simulink model "learning"  (R2021a)
settings: Solver=VariableStepAuto  StartTime=0.0  StopTime=1.5  RelTol=1e-3
undefined symbols (not defined in the file): Radix
libraries: dspswit3 x4, dspxfrm3 x3, dspstat3 x2, visionstatistics x1, dspindex x1, dspsigops x1
settings Model: Creator=DAO1WA2  LastModifiedBy=O Darwish
settings SolverCC: AlgebraicLoopSolver=TrustRegion
settings DebuggingCC: SFMachineParentedDataDiag=warning

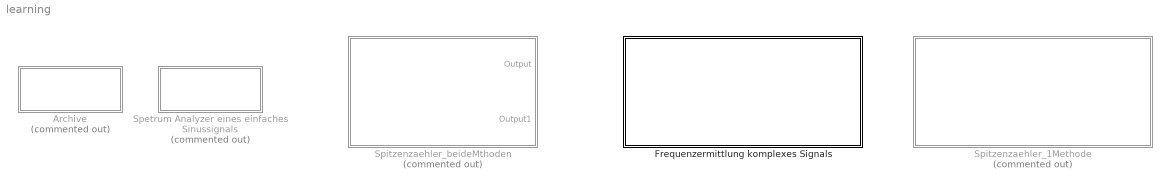
== system learning ==
  Archive : Subsystem  Commented=on
  Frequenzermittlung komplexes Signals : Subsystem
  Spetrum Analyzer eines einfaches Sinussignals : Subsystem  Commented=on
  Spitzenzaehler_1Methode : Subsystem  Commented=on
  Spitzenzaehler_beideMthoden : Subsystem  Commented=on

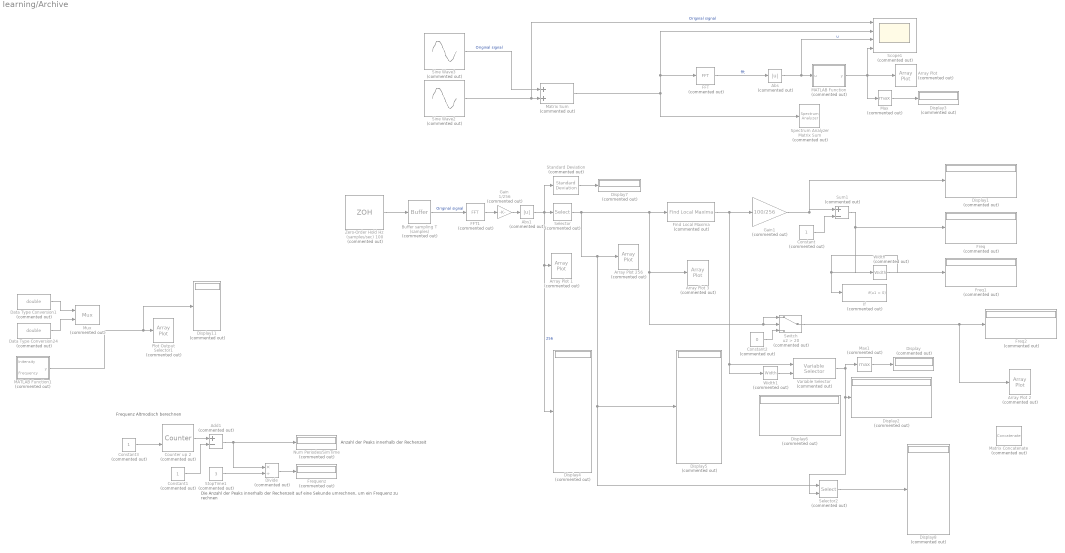
== system learning/Archive ==
  note: Frequenz Altmodisch berechnen
  note: Die Anzahl der Peaks innerhalb der Rechenzeit auf eine Sekunde umrechnen, um ein Frequenz zu rechnen
  note: Anzahl der Peaks innerhalb der Rechenzeit
  Abs : Abs  Commented=on
  Abs1 : Abs  Commented=on
  Add1 : Sum  Commented=on  Inputs=+-
  Array Plot : ArrayPlot  Commented=on  WindowPosition=[1925.8 897 1920 1095.2]  AxesScaling=Manual  YLimits=[89.0635,109.063]  ShowLegend=on  DefaultConfigurationName=dsp.scopes.ArrayPlotBlockSpecification
  Array Plot 1 : ArrayPlot  Commented=on  WindowPosition=[1.8 32.2 1532.8 748.8]  AxesScaling=Manual  YLimits=[-12.1535,116.039]  DefaultConfigurationName=dsp.scopes.ArrayPlotBlockSpecification
  Array Plot 2 : ArrayPlot  Commented=on  WindowPosition=[2 32.2 1532.8 748.8]  AxesScaling=Manual  YLimits=[-11.2764,109.153]  DefaultConfigurationName=dsp.scopes.ArrayPlotBlockSpecification
  Array Plot 256 : ArrayPlot  Commented=on  WindowPosition=[1.8 32.2 1532.8 748.8]  AxesScaling=Manual  YLimits=[-11.2764,109.153]  DefaultConfigurationName=dsp.scopes.ArrayPlotBlockSpecification
  Array Plot 3 : ArrayPlot  Commented=on  WindowPosition=[2.6 33 1532.8 748.8]  AxesScaling=Manual  YLimits=[-11.2764,109.153]  DefaultConfigurationName=dsp.scopes.ArrayPlotBlockSpecification
  Buffer sampling T (samples) : Buffer  Commented=on  N=256  V=128  OutputFrames=off
  Constant : Constant  Commented=on
  Constant1 : Constant  Commented=on
  Constant2 : Constant  Commented=on  Value=0
  Constant3 : Constant  Commented=on
  Counter up 2 : dspswit3/Counter  Commented=on  Direction=Up  CountEvent=Rising edge  CounterSize=User defined  MaxCount=255  InitialCount=0  Output=Count  HitValue=32  ResetInput=on  SamplesPerFrame=1  Ts=1  CntDtype=double  HitDtype=Logical
  Data Type Conversion1 : DataTypeConversion  Commented=on  OutDataTypeStr=double  RndMeth=Zero
  Data Type Conversion24 : DataTypeConversion  Commented=on  OutDataTypeStr=double  RndMeth=Zero
  Display{,1..8,11} (10 alike) : Display  Commented=on
  Divide : Product  Commented=on  Inputs=*/
  FFT : dspxfrm3/FFT  Commented=on  FFTImplementation=Auto  CompMethod=Table lookup  TableOpt=NEW  TableOptActive=Speed  BitRevOrder=off  Normalize=on  InheritFFTLength=on  FFTLength=64  WrapInput=on  roundingMode=Floor  overflowMode=off  firstCoeffDataTypeStr=Inherit: Same word length as input  firstCoeffLastDataTypeStr=Inherit: Same word length as input  outputMin=[]  outputMax=[]
  FFT1 : dspxfrm3/FFT  Commented=on  FFTImplementation=Radix-2  CompMethod=Table lookup  TableOpt=NEW  TableOptActive=Speed  BitRevOrder=off  Normalize=off  InheritFFTLength=on  FFTLength=256  WrapInput=off  roundingMode=Floor  overflowMode=off  firstCoeffDataTypeStr=Inherit: Same word length as input  firstCoeffLastDataTypeStr=Inherit: Same word length as input  outputMin=[]  outputMax=[]
  Find Local Maxima : visionstatistics/Find Local Maxima  Commented=on  num_peaks=4  nhood_size=[9 1]  src_thresh=Obsolete9b  src_thresh_inuse=Specify via dialog  threshold=10  inputIsHough=off  dt_peak=double  isOutVarDim=on  dt_count=double
      settings: SourceProductBaseCode=VP
  Freq : Display  Commented=on
  Freq1 : Display  Commented=on
  Freq2 : Display  Commented=on
  Frequenz : Display  Commented=on
  Gain : Gain  Commented=on  Gain=1/256
  Gain1 : Gain  Commented=on  Gain=100/256
  If : If  Commented=on  ShowElse=off
  MATLAB Function : MATLAB Function  Commented=on  TreatAsAtomicUnit=on
  MATLAB Function1 : MATLAB Function  Commented=on  TreatAsAtomicUnit=on
  Matrix Concatenate : Concatenate  Commented=on  NumInputs=1  Mode=Multidimensional array
  Matrix Sum : Sum  Commented=on
  Max : MinMax  Commented=on  Function=max
  Max1 : MinMax  Commented=on  Function=max
  Mux : Mux  Commented=on  Inputs=2
      settings: DisplayOption=signals
  Num Periodes/SimTime : Display  Commented=on
  Plot Output Selector1 : ArrayPlot  Commented=on  WindowPosition=[1 31.4 1536 758.4]  AxesScaling=Manual  YLimits=[-12.0102,109.123]  DefaultConfigurationName=dsp.scopes.ArrayPlotBlockSpecification
  Scope1 : Scope  Commented=on  NumInputPorts=4
  Selector : Selector  Commented=on  IndexOptions=Index vector (dialog)  Indices=1:128  OutputSizes=1
  Selector2 : Selector  Commented=on  IndexMode=Zero-based  IndexOptions=Index vector (port)  Indices=[1 3]  OutputSizes=1
  Sine Wave2 : Sin  Commented=on  Amplitude=325  Frequency=200  Samples=100  SampleTime=0.0001
  Sine Wave3 : Sin  Commented=on  SineType=Sample based  Amplitude=325  Frequency=314  Samples=100  SampleTime=0.0001
  Spectrum Analyzer Matrix Sum : SpectrumAnalyzer  Commented=on
  Standard Deviation : dspstat3/Standard Deviation  Commented=on  run=off  directionMode=Each column  dimension=1  InputProcessing=Columns as channels (frame based)  reset_popup=None  roiEnable=off  roiType=Rectangles  roiPortion=Entire ROI  roiOutput=Individual statistics for each ROI  roiFlag=off
      settings: SourceProductBaseCode=DS
  StopTime1 : Constant  Commented=on  Value=3
  Sum1 : Sum  Commented=on  Inputs=|+-
  Switch : Switch  Commented=on  Criteria=u2 > Threshold  Threshold=20
  Variable Selector : dspindex/Variable Selector  Commented=on  NumInputs=1  rowsOrCols=Columns  IdxMode=Variable  Elements=[1 3]  ZerOneIdxMode=One-based  errmode=Clip Index  FillMode=off  FillValues=0
  Width : Width  Commented=on
  Width1 : Width  Commented=on
  Zero-Order Hold Hz (samples/sec) 100 : ZeroOrderHold  Commented=on  SampleTime=1e-2
  wires:
  FFT/1 -> Abs/1  "fft"
  MATLAB Function1/1(y) -> Display11/1, Plot Output Selector1/1
  Divide/1 -> Frequenz/1
  Gain1/1 -> Display1/1, Sum1/1
  Selector/1 -> Find Local Maxima/1, Array Plot 3/1, Switch/1, Switch/2, Display5/1, Selector2/1, Array Plot 256/1
  Standard Deviation/1 -> Display7/1
  Constant2/1 -> Switch/3
  MATLAB Function/1(y) -> Scope1/4, Max/1, Array Plot/1
  Data Type Conversion1/1 -> Mux/1
  Width1/1 -> Variable Selector/2
  Switch/1 -> Array Plot 2/1, Freq2/1
  Max/1 -> Display3/1
  Sum1/1 -> Width/1, Freq/1
  Max1/1 -> Display/1
  Width/1 -> If/1, Freq1/1
  Constant/1 -> Sum1/2
  Variable Selector/1 -> Selector2/2, Display2/1, Max1/1
  Abs1/1 -> Array Plot 1/1, Display4/1, Standard Deviation/1, Selector/1  "256"
  Gain/1 -> Abs1/1
  Buffer sampling T (samples)/1 -> FFT1/1  "Original signal"
  FFT1/1 -> Gain/1
  Selector2/1 -> Display8/1
  Find Local Maxima/1 -> Width1/1, Variable Selector/1, Gain1/1
  Data Type Conversion24/1 -> Mux/2
  Constant1/1 -> Add1/2
  Zero-Order Hold Hz (samples/sec) 100/1 -> Buffer sampling T (samples)/1
  Sine Wave3/1 -> Matrix Sum/1  "Original signal"
  Add1/1 -> Divide/1, Num Periodes/SimTime/1
  Abs/1 -> Scope1/3, MATLAB Function/1(u)  "u"
  StopTime1/1 -> Divide/2
  Counter up 2/1 -> Add1/1
  Matrix Sum/1 -> FFT/1, Scope1/2, Spectrum Analyzer Matrix Sum/1
  Constant3/1 -> Counter up 2/2
  Sine Wave2/1 -> Scope1/1, Matrix Sum/2  "Original signal"

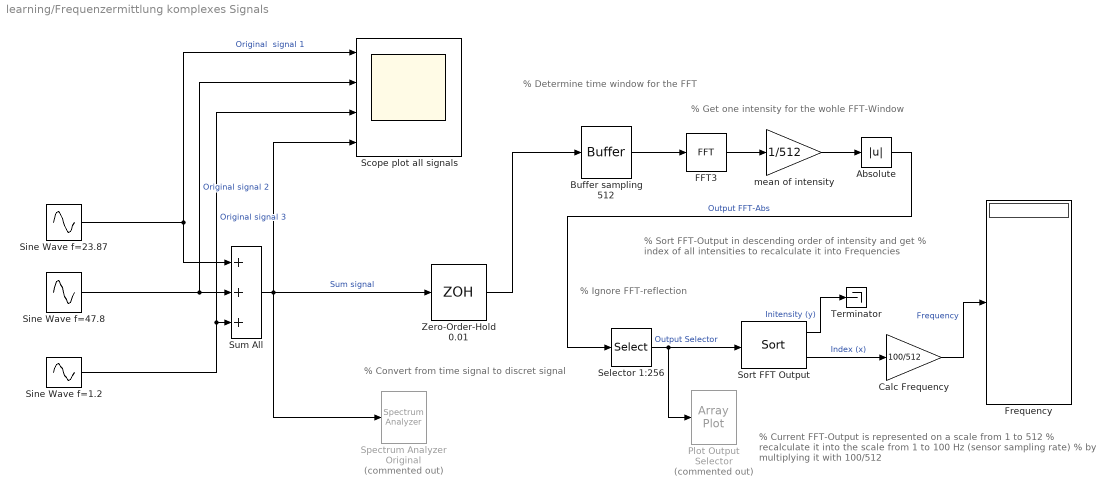
== system learning/Frequenzermittlung komplexes Signals ==
  note: % Get one intensity for the wohle FFT-Window
  note: % Determine time window for the FFT
  note: % Convert from time signal to discret signal
  note: % Ignore FFT-reflection
  note: % Sort FFT-Output in descending order of intensity and get
      | % index of all intensities to recalculate it into Frequencies
  note: % Current FFT-Output is represented on a scale from 1 to 512
      | % recalculate it into the scale from 1 to 100 Hz (sensor sampling rate)
      | % by multiplying it with 100/512
  Absolute : Abs
  Buffer sampling 512 : Buffer  N=512  OutputFrames=off
  Calc Frequency : Gain  Gain=100/512
  FFT3 : dspxfrm3/FFT  FFTImplementation=Radix-2  CompMethod=Table lookup  TableOpt=NEW  TableOptActive=Speed  BitRevOrder=off  Normalize=off  InheritFFTLength=on  FFTLength=64  WrapInput=on  roundingMode=Floor  overflowMode=off  firstCoeffDataTypeStr=Inherit: Same word length as input  firstCoeffLastDataTypeStr=Inherit: Same word length as input  outputMin=[]  outputMax=[]
  Frequency : Display
  Plot Output Selector : ArrayPlot  Commented=on  WindowPosition=[1.000000,31.000000,1536.000000,758.000000,]  AxesScaling=Manual  YLimits=[-12.0102,109.123]  DefaultConfigurationName=dsp.scopes.ArrayPlotBlockSpecification
  Scope plot all signals : Scope  NumInputPorts=4
  Selector 1:256 : Selector  IndexMode=Zero-based  IndexOptions=Index vector (dialog)  Indices=1:256  OutputSizes=1
  Sine Wave f=1.2 : Sin  Amplitude=200  Frequency=7  Samples=100  SampleTime=0.00001
  Sine Wave f=23.87 : Sin  Amplitude=200  Frequency=150  Samples=100  SampleTime=0.00001
  Sine Wave f=47.8 : Sin  Amplitude=200  Frequency=300  Samples=100  SampleTime=0.00001
  Sort FFT Output : dspstat3/Sort  otype=Value and Index  dir=Descending  sortAlg=Quick sort  roundingMode=Floor  overflowMode=off  accumDataTypeStr=Inherit: Same as product output  accumLastDataTypeStr=Inherit: Same as product output
      settings: SourceProductBaseCode=DS
  Spectrum Analyzer Original : SpectrumAnalyzer  Commented=on
  Sum All : Sum  Inputs=+++
  Terminator : Terminator
  Zero-Order-Hold 0.01 : ZeroOrderHold  SampleTime=0.01
  mean of intensity : Gain  Gain=1/512
  wires:
  Absolute/1 -> Selector 1:256/1  "Output FFT-Abs"
  Sine Wave f=47.8/1 -> Scope plot all signals/2, Sum All/2  "Original signal 2"
  Sum All/1 -> Scope plot all signals/4, Zero-Order-Hold 0.01/1, Spectrum Analyzer Original/1  "Sum signal"
  Zero-Order-Hold 0.01/1 -> Buffer sampling 512/1
  Sine Wave f=1.2/1 -> Scope plot all signals/3, Sum All/3  "Original signal 3"
  Buffer sampling 512/1 -> FFT3/1
  FFT3/1 -> mean of intensity/1
  Sort FFT Output/1 -> Terminator/1  "Initensity (y)"
  Calc Frequency/1 -> Frequency/1  "Frequency"
  Sort FFT Output/2 -> Calc Frequency/1  "Index (x)"
  Selector 1:256/1 -> Sort FFT Output/1, Plot Output Selector/1  "Output Selector"
  Sine Wave f=23.87/1 -> Scope plot all signals/1, Sum All/1  "Original  signal 1"
  mean of intensity/1 -> Absolute/1

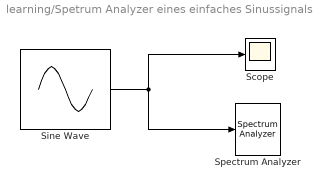
== system learning/Spetrum Analyzer eines einfaches Sinussignals ==
  Scope : Scope
  Sine Wave : Sin  SineType=Sample based  Amplitude=325  Samples=100  SampleTime=0.0001
  Spectrum Analyzer : SpectrumAnalyzer
  wires:
  Sine Wave/1 -> Scope/1, Spectrum Analyzer/1

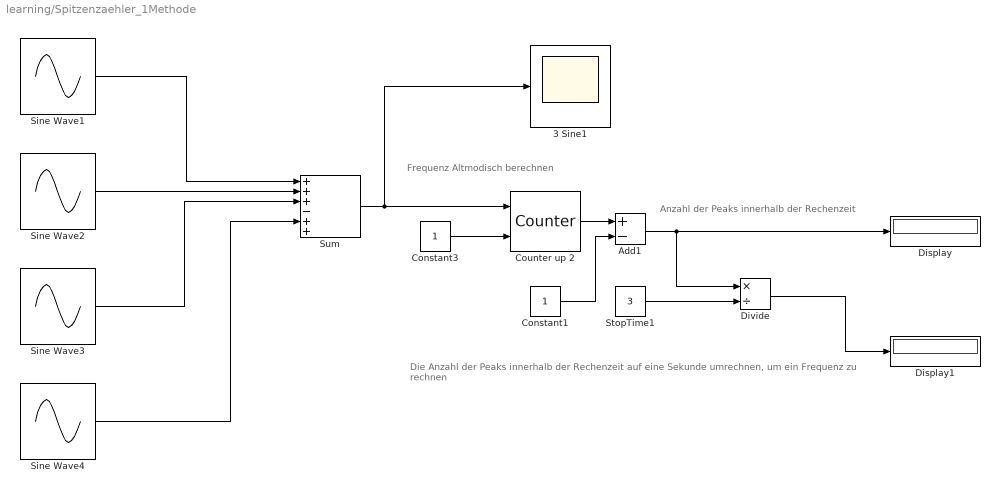
== system learning/Spitzenzaehler_1Methode ==
  note: Frequenz Altmodisch berechnen
  note: Anzahl der Peaks innerhalb der Rechenzeit
  note: Die Anzahl der Peaks innerhalb der Rechenzeit auf eine Sekunde umrechnen, um ein Frequenz zu rechnen
  3 Sine1 : Scope
  Add1 : Sum  Inputs=+-
  Constant1 : Constant
  Constant3 : Constant
  Counter up 2 : dspswit3/Counter  Direction=Up  CountEvent=Either edge  CounterSize=User defined  MaxCount=255  InitialCount=0  Output=Count  HitValue=32  ResetInput=on  SamplesPerFrame=1  Ts=1  CntDtype=double  HitDtype=Logical
  Display : Display
  Display1 : Display
  Divide : Product  Inputs=*/
  Sine Wave1 : Sin  Amplitude=20  Frequency=50  SampleTime=0.0001
  Sine Wave2 : Sin  Amplitude=20  Frequency=20  SampleTime=0.0001
  Sine Wave3 : Sin  Amplitude=20  Frequency=5  SampleTime=0.0001
  Sine Wave4 : Sin  Amplitude=20  Frequency=100  SampleTime=0.0001
  StopTime1 : Constant  Value=3
  Sum : Sum  Inputs=+++-++
  wires:
  Constant1/1 -> Add1/2
  Constant3/1 -> Counter up 2/2
  Divide/1 -> Display1/1
  Add1/1 -> Display/1, Divide/1
  StopTime1/1 -> Divide/2
  Sine Wave3/1 -> Sum/3
  Sum/1 -> 3 Sine1/1, Counter up 2/1
  Sine Wave4/1 -> Sum/5
  Sine Wave1/1 -> Sum/1
  Sine Wave2/1 -> Sum/2
  Counter up 2/1 -> Add1/1

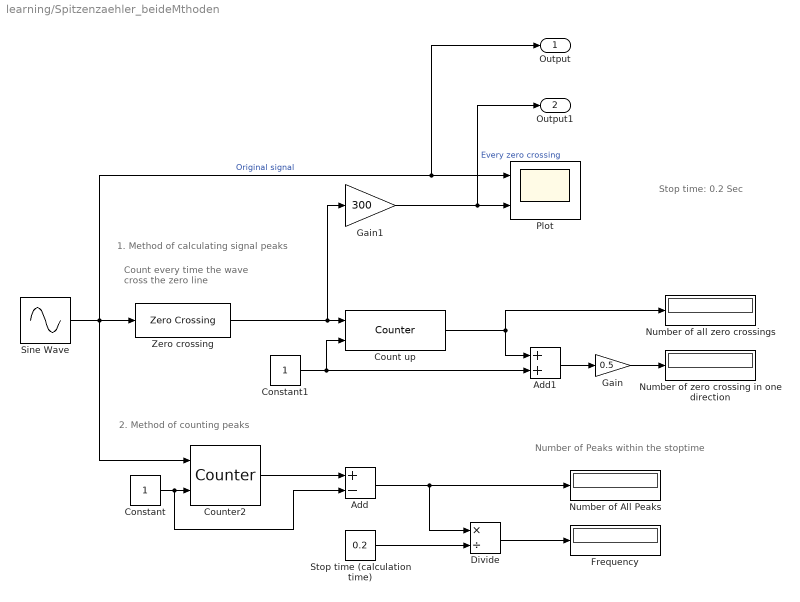
== system learning/Spitzenzaehler_beideMthoden ==
  note: 2. Method of counting peaks
  note: 1. Method of calculating signal peaks
  note: Number of Peaks within the stoptime
  note: Stop time: 0.2 Sec
  note: Count every time the wave
      | cross the zero line
  Add : Sum  Inputs=+-
  Add1 : Sum
  Constant : Constant
  Constant1 : Constant
  Count up : dspswit3/Counter  Direction=Up  CountEvent=Rising edge  CounterSize=User defined  MaxCount=255  InitialCount=0  Output=Count  HitValue=32  ResetInput=on  SamplesPerFrame=1  Ts=1  CntDtype=double  HitDtype=Logical
  Counter2 : dspswit3/Counter  Direction=Up  CountEvent=Rising edge  CounterSize=User defined  MaxCount=255  InitialCount=0  Output=Count  HitValue=32  ResetInput=on  SamplesPerFrame=1  Ts=1  CntDtype=double  HitDtype=Logical
  Divide : Product  Inputs=*/
  Frequency : Display
  Gain : Gain  Gain=0.5
  Gain1 : Gain  Gain=300
  Number of All Peaks : Display
  Number of all zero crossings : Display
  Number of zero crossing in one direction : Display
  "Plot " : Scope  NumInputPorts=2
  "Sine Wave " : Sin  Amplitude=325  Frequency=620  Samples=5  SampleTime=0.00001
  Stop time (calculation time) : Constant  Value=0.2
  "Zero crossing " : dspsigops/Zero Crossing  InputProcessing=Columns as channels (frame based)
      settings: SourceProductBaseCode=DS
  Output : Outport
  Output1 : Outport  Port=2
  wires:
  Add/1 -> Divide/1, Number of All Peaks/1
  Constant/1 -> Add/2, Counter2/2
  "Sine Wave "/1 -> Output/1, "Plot "/1, Counter2/1, "Zero crossing "/1  "Original signal"
  Gain1/1 -> Output1/1, "Plot "/2  "Every zero crossing"
  Stop time (calculation time)/1 -> Divide/2
  Divide/1 -> Frequency/1
  Gain/1 -> Number of zero crossing in one direction/1
  Count up/1 -> Number of all zero crossings/1, Add1/1
  Counter2/1 -> Add/1
  "Zero crossing "/1 -> Count up/1, Gain1/1
  Constant1/1 -> Add1/2, Count up/2
  Add1/1 -> Gain/1

== matlab function learning/Archive/MATLAB Function ==
  data: u input; y output
function y = fcn(u)
y = fftshift(u);
end

== matlab function learning/Archive/MATLAB Function1 ==
  data: Initensity input; y output; Frequency input
function y = fcn(Initensity, Frequency)

% Initensity = Initensity (1:10);
% Frequency = Frequency (1:10);
y = zeros(length(Initensity), 2);
y(:,1) = Frequency; 
y(:, 2) = Initensity;


1;
